simulink model "CF025A_GmFctDiArbn"  (R2013b)
settings: Solver=FixedStepDiscrete  SolverMode=SingleTasking  StartTime=0.0  StopTime=60  FixedStep=0.002  RelTol=1e-3
values from neighbouring files (symbols this model uses):
  GmFctDiArbnEotHwAgThd = DataDict.Calibration    [CF025A_GmFctDiArbn_DataDict.m]
  GmFctDiArbnEotTi = DataDict.Calibration    [CF025A_GmFctDiArbn_DataDict.m]
  GmFctDiArbnOnCentrHwAgThd = DataDict.Calibration    [CF025A_GmFctDiArbn_DataDict.m]
  GmFctDiArbnOnCentrHwTqThd = DataDict.Calibration    [CF025A_GmFctDiArbn_DataDict.m]
  GmFctDiArbnOnCentrTi = DataDict.Calibration    [CF025A_GmFctDiArbn_DataDict.m]
  GmFctDiArbnSrvTi = DataDict.Calibration    [CF025A_GmFctDiArbn_DataDict.m]
  MICROSECTOSEC_ULS_F32 = DataDict.Constant    [CF025A_GmFctDiArbn_DataDict.m]
  ZEROHWAG_HWDEG_F32 = DataDict.Constant    [CF025A_GmFctDiArbn_DataDict.m]
undefined symbols (not defined in the file or in its folder): GmFctDiArbnSts1, LoaSt1
libraries: simulink x7, FixdToFloat x4
(part 3 of 3)

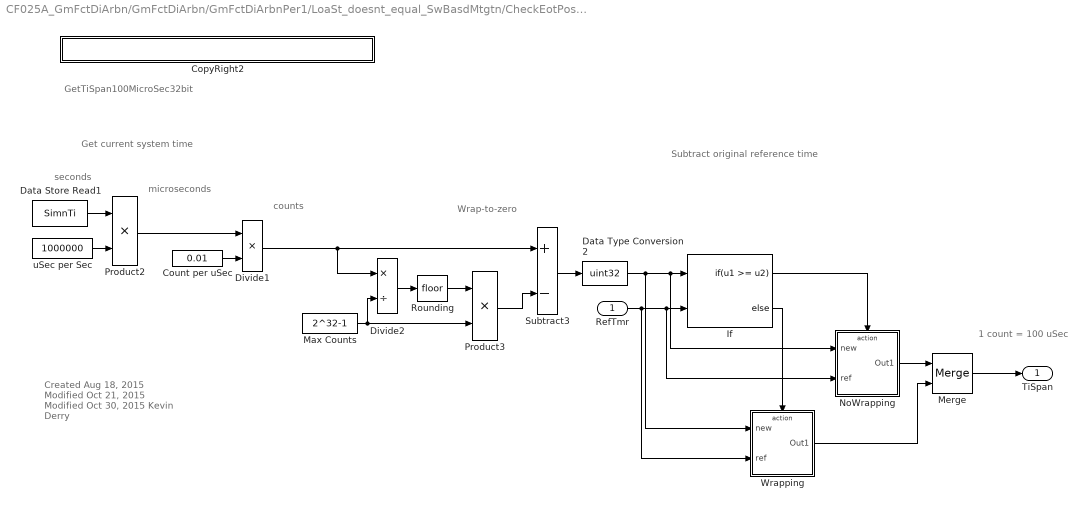
== system CF025A_GmFctDiArbn/GmFctDiArbn/GmFctDiArbnPer1/LoaSt_doesnt_equal_SwBasdMtgtn/CheckEotPosInRange/InProc/InRangeCwDirection/InCwEotElpdTi/ElpdTi_Check/GetTiSpan100MicroSec32bit ==
  note: Created Aug 18, 2015
      | Modified Oct 21, 2015
      | Modified Oct 30, 2015
      | Kevin Derry
  note: GetTiSpan100MicroSec32bit
  note: Get current system time
  note: 1 count = 100 uSec
  note: Wrap-to-zero
  note: counts
  note: microseconds
  note: seconds
  note: Subtract original reference time
  RefTmr : Inport
  CopyRight2 : Subsystem  Description=|  mask(Copyright Information){none=on}
      | Copyright info block.                                               
      |                                                                     
      | Place copyright information at the top of every subsystem in design.
      mask prompts: none "No parameters"
      mask help: Place copyright information at the top of every subsystem in design.
      mask Display:
      | NxtrConf = 'Nexteer Confidential';
      | 
      | sys = bdroot; %handle for the current model ("system")
      | first = get_param(sys,'Created');
      | if(isempty(first))
      |     first = datestr(now,'yyyy');
      | else
      |     first = first(end-3:end);  %year is last four digits
      | end
      | 
      | last = get_param(sys,'LastModifiedDate');
      | if isempty(last)
      |     last = datestr(now,'yyyy');
      | else
      |     last = last(end-3:end);
      | end
      | 
      | if strcmp(first,last)
      |     fprintf('%s -- Copyright %s Nexteer',NxtrConf,first)
      | else
      |     fprintf('%s -- %s%s- %s Nexteer',NxtrConf,char(169),first,last)
      | end
  Count per uSec : Constant  Value=0.01
  Data Store Read1 : DataStoreRead  DataStoreName=SimnTi
  Data Type Conversion2 : DataTypeConversion  OutDataTypeStr=uint32
  Divide1 : Product  Inputs=**
  Divide2 : Product  Inputs=*/
  If : If  NumInputs=2  IfExpression=u1 >= u2
  Max Counts : Constant  Value=2^32-1
  Merge : Merge
  NoWrapping : Subsystem  TreatAsAtomicUnit=on
  Product2 : Product
  Product3 : Product
  Rounding : Rounding
  Subtract3 : Sum  Inputs=+-
  Wrapping : Subsystem  TreatAsAtomicUnit=on
  uSec per Sec : Constant  Value=1000000
  TiSpan : Outport
  wires:
  Data Type Conversion2/1 -> Wrapping/1(new), NoWrapping/1(new), If/1
  RefTmr/1 -> Wrapping/2(ref), NoWrapping/2(ref), If/2
  Merge/1 -> TiSpan/1
  uSec per Sec/1 -> Product2/2
  Count per uSec/1 -> Divide1/2
  Data Store Read1/1 -> Product2/1
  Product2/1 -> Divide1/1
  Divide1/1 -> Subtract3/1, Divide2/1
  Max Counts/1 -> Product3/2, Divide2/2
  Divide2/1 -> Rounding/1
  Rounding/1 -> Product3/1
  Subtract3/1 -> Data Type Conversion2/1
  Product3/1 -> Subtract3/2
  If/1 -> NoWrapping/Action
  If/2 -> Wrapping/Action
  NoWrapping/1(Out1) -> Merge/1
  Wrapping/1(Out1) -> Merge/2

== system CF025A_GmFctDiArbn/GmFctDiArbn/GmFctDiArbnPer1/LoaSt_doesnt_equal_SwBasdMtgtn/CheckEotPosInRange/InProc/InRangeCwDirection/InCwEotElpdTi/ElpdTi_Start/Copyright1 ==

== system CF025A_GmFctDiArbn/GmFctDiArbn/GmFctDiArbnPer1/LoaSt_doesnt_equal_SwBasdMtgtn/CheckEotPosInRange/InProc/InRangeCwDirection/InCwEotElpdTi/ElpdTi_Start/GetRefTmr100MicroSec32bit ==
  note: 1 count = 100 uSec
  note: seconds
  note: microseconds
  note: counts
  note: Wrap-to-zero
  note: GetRefTmr100MicroSec32bit
  note: Created Aug 18, 2015
      | Modified Oct 21, 2015
      | Modified Oct 30, 2015
      | Kevin Derry
  CopyRight2 : Subsystem  Description=|  mask(Copyright Information){none=on}
      | Copyright info block.                                               
      |                                                                     
      | Place copyright information at the top of every subsystem in design.
      mask prompts: none "No parameters"
      mask help: Place copyright information at the top of every subsystem in design.
      mask Display:
      | NxtrConf = 'Nexteer Confidential';
      | 
      | sys = bdroot; %handle for the current model ("system")
      | first = get_param(sys,'Created');
      | if(isempty(first))
      |     first = datestr(now,'yyyy');
      | else
      |     first = first(end-3:end);  %year is last four digits
      | end
      | 
      | last = get_param(sys,'LastModifiedDate');
      | if isempty(last)
      |     last = datestr(now,'yyyy');
      | else
      |     last = last(end-3:end);
      | end
      | 
      | if strcmp(first,last)
      |     fprintf('%s -- Copyright %s Nexteer',NxtrConf,first)
      | else
      |     fprintf('%s -- %s%s- %s Nexteer',NxtrConf,char(169),first,last)
      | end
  Count per uSec : Constant  Value=0.01
  Data Store Read1 : DataStoreRead  DataStoreName=SimnTi
  Data Type Conversion1 : DataTypeConversion  OutDataTypeStr=uint32
  Divide1 : Product  Inputs=**
  Divide2 : Product  Inputs=*/
  Max Counts : Constant  Value=2^32-1
  Product1 : Product
  Product2 : Product
  Rounding : Rounding
  Subtract1 : Sum  Inputs=+-
  uSec per Sec : Constant  Value=1000000
  RefTmr : Outport
  wires:
  Product2/1 -> Subtract1/2
  Subtract1/1 -> Data Type Conversion1/1
  Rounding/1 -> Product2/1
  Divide2/1 -> Rounding/1
  Max Counts/1 -> Divide2/2, Product2/2
  Divide1/1 -> Divide2/1, Subtract1/1
  Product1/1 -> Divide1/1
  Count per uSec/1 -> Divide1/2
  uSec per Sec/1 -> Product1/2
  Data Type Conversion1/1 -> RefTmr/1
  Data Store Read1/1 -> Product1/1

== system CF025A_GmFctDiArbn/GmFctDiArbn/GmFctDiArbnPer1/LoaSt_doesnt_equal_SwBasdMtgtn/CheckEotPosInRange/InProc/InRangeCwDirection/InCwEotElpdTi/ElpdTi_Zero/Copyright1 ==

== system CF025A_GmFctDiArbn/GmFctDiArbn/GmFctDiArbnPer1/LoaSt_doesnt_equal_SwBasdMtgtn/CheckHwTqZeroAndHwAgZero/IfBothEotElpdTimeMet/OnCentrElpdTi/ElpdTi_Check/GetTiSpan100MicroSec32bit/CopyRight2 ==

== system CF025A_GmFctDiArbn/GmFctDiArbn/GmFctDiArbnPer1/LoaSt_doesnt_equal_SwBasdMtgtn/CheckHwTqZeroAndHwAgZero/IfBothEotElpdTimeMet/OnCentrElpdTi/ElpdTi_Check/GetTiSpan100MicroSec32bit/NoWrapping ==
  new : Inport
  ref : Inport  Port=2
  Action Port : ActionPort  ActionType=then
  CopyRight2 : Subsystem  Description=|  mask(Copyright Information){none=on}
      | Copyright info block.                                               
      |                                                                     
      | Place copyright information at the top of every subsystem in design.
      mask prompts: none "No parameters"
      mask help: Place copyright information at the top of every subsystem in design.
      mask Display:
      | NxtrConf = 'Nexteer Confidential';
      | 
      | sys = bdroot; %handle for the current model ("system")
      | first = get_param(sys,'Created');
      | if(isempty(first))
      |     first = datestr(now,'yyyy');
      | else
      |     first = first(end-3:end);  %year is last four digits
      | end
      | 
      | last = get_param(sys,'LastModifiedDate');
      | if isempty(last)
      |     last = datestr(now,'yyyy');
      | else
      |     last = last(end-3:end);
      | end
      | 
      | if strcmp(first,last)
      |     fprintf('%s -- Copyright %s Nexteer',NxtrConf,first)
      | else
      |     fprintf('%s -- %s%s- %s Nexteer',NxtrConf,char(169),first,last)
      | end
  Subtract1 : Sum  Inputs=+-
  Out1 : Outport
  wires:
  Subtract1/1 -> Out1/1
  new/1 -> Subtract1/1
  ref/1 -> Subtract1/2

== system CF025A_GmFctDiArbn/GmFctDiArbn/GmFctDiArbnPer1/LoaSt_doesnt_equal_SwBasdMtgtn/CheckHwTqZeroAndHwAgZero/IfBothEotElpdTimeMet/OnCentrElpdTi/ElpdTi_Check/GetTiSpan100MicroSec32bit/Wrapping ==
  new : Inport
  ref : Inport  Port=2
  Action Port : ActionPort  ActionType=else
  CopyRight2 : Subsystem  Description=|  mask(Copyright Information){none=on}
      | Copyright info block.                                               
      |                                                                     
      | Place copyright information at the top of every subsystem in design.
      mask prompts: none "No parameters"
      mask help: Place copyright information at the top of every subsystem in design.
      mask Display:
      | NxtrConf = 'Nexteer Confidential';
      | 
      | sys = bdroot; %handle for the current model ("system")
      | first = get_param(sys,'Created');
      | if(isempty(first))
      |     first = datestr(now,'yyyy');
      | else
      |     first = first(end-3:end);  %year is last four digits
      | end
      | 
      | last = get_param(sys,'LastModifiedDate');
      | if isempty(last)
      |     last = datestr(now,'yyyy');
      | else
      |     last = last(end-3:end);
      | end
      | 
      | if strcmp(first,last)
      |     fprintf('%s -- Copyright %s Nexteer',NxtrConf,first)
      | else
      |     fprintf('%s -- %s%s- %s Nexteer',NxtrConf,char(169),first,last)
      | end
  Max Counts : Constant  Value=2^32-1  OutDataTypeStr=uint32
  Subtract1 : Sum  Inputs=+-+
  Out1 : Outport
  wires:
  Subtract1/1 -> Out1/1
  Max Counts/1 -> Subtract1/1
  ref/1 -> Subtract1/2
  new/1 -> Subtract1/3

== system CF025A_GmFctDiArbn/GmFctDiArbn/GmFctDiArbnPer1/LoaSt_doesnt_equal_SwBasdMtgtn/CheckHwTqZeroAndHwAgZero/IfBothEotElpdTimeMet/OnCentrElpdTi/ElpdTi_Start/GetRefTmr100MicroSec32bit/CopyRight2 ==

== system CF025A_GmFctDiArbn/GmFctDiArbn/GmFctDiArbnPer1/LoaSt_doesnt_equal_SwBasdMtgtn/CheckEotPosInRange/InProc/InRangeCcwDirection/InCcwEotElpdTi/ElpdTi_Check/GetTiSpan100MicroSec32bit/CopyRight2 ==

== system CF025A_GmFctDiArbn/GmFctDiArbn/GmFctDiArbnPer1/LoaSt_doesnt_equal_SwBasdMtgtn/CheckEotPosInRange/InProc/InRangeCcwDirection/InCcwEotElpdTi/ElpdTi_Check/GetTiSpan100MicroSec32bit/NoWrapping ==
  new : Inport
  ref : Inport  Port=2
  Action Port : ActionPort  ActionType=then
  CopyRight2 : Subsystem  Description=|  mask(Copyright Information){none=on}
      | Copyright info block.                                               
      |                                                                     
      | Place copyright information at the top of every subsystem in design.
      mask prompts: none "No parameters"
      mask help: Place copyright information at the top of every subsystem in design.
      mask Display:
      | NxtrConf = 'Nexteer Confidential';
      | 
      | sys = bdroot; %handle for the current model ("system")
      | first = get_param(sys,'Created');
      | if(isempty(first))
      |     first = datestr(now,'yyyy');
      | else
      |     first = first(end-3:end);  %year is last four digits
      | end
      | 
      | last = get_param(sys,'LastModifiedDate');
      | if isempty(last)
      |     last = datestr(now,'yyyy');
      | else
      |     last = last(end-3:end);
      | end
      | 
      | if strcmp(first,last)
      |     fprintf('%s -- Copyright %s Nexteer',NxtrConf,first)
      | else
      |     fprintf('%s -- %s%s- %s Nexteer',NxtrConf,char(169),first,last)
      | end
  Subtract1 : Sum  Inputs=+-
  Out1 : Outport
  wires:
  ref/1 -> Subtract1/2
  new/1 -> Subtract1/1
  Subtract1/1 -> Out1/1

== system CF025A_GmFctDiArbn/GmFctDiArbn/GmFctDiArbnPer1/LoaSt_doesnt_equal_SwBasdMtgtn/CheckEotPosInRange/InProc/InRangeCcwDirection/InCcwEotElpdTi/ElpdTi_Check/GetTiSpan100MicroSec32bit/Wrapping ==
  new : Inport
  ref : Inport  Port=2
  Action Port : ActionPort  ActionType=else
  CopyRight2 : Subsystem  Description=|  mask(Copyright Information){none=on}
      | Copyright info block.                                               
      |                                                                     
      | Place copyright information at the top of every subsystem in design.
      mask prompts: none "No parameters"
      mask help: Place copyright information at the top of every subsystem in design.
      mask Display:
      | NxtrConf = 'Nexteer Confidential';
      | 
      | sys = bdroot; %handle for the current model ("system")
      | first = get_param(sys,'Created');
      | if(isempty(first))
      |     first = datestr(now,'yyyy');
      | else
      |     first = first(end-3:end);  %year is last four digits
      | end
      | 
      | last = get_param(sys,'LastModifiedDate');
      | if isempty(last)
      |     last = datestr(now,'yyyy');
      | else
      |     last = last(end-3:end);
      | end
      | 
      | if strcmp(first,last)
      |     fprintf('%s -- Copyright %s Nexteer',NxtrConf,first)
      | else
      |     fprintf('%s -- %s%s- %s Nexteer',NxtrConf,char(169),first,last)
      | end
  Max Counts : Constant  Value=2^32-1  OutDataTypeStr=uint32
  Subtract1 : Sum  Inputs=+-+
  Out1 : Outport
  wires:
  new/1 -> Subtract1/3
  ref/1 -> Subtract1/2
  Max Counts/1 -> Subtract1/1
  Subtract1/1 -> Out1/1

== system CF025A_GmFctDiArbn/GmFctDiArbn/GmFctDiArbnPer1/LoaSt_doesnt_equal_SwBasdMtgtn/CheckEotPosInRange/InProc/InRangeCcwDirection/InCcwEotElpdTi/ElpdTi_Start/GetRefTmr100MicroSec32bit/CopyRight2 ==

== system CF025A_GmFctDiArbn/GmFctDiArbn/GmFctDiArbnPer1/LoaSt_doesnt_equal_SwBasdMtgtn/CheckEotPosInRange/InProc/InRangeCwDirection/InCwEotElpdTi/ElpdTi_Check/GetTiSpan100MicroSec32bit/CopyRight2 ==

== system CF025A_GmFctDiArbn/GmFctDiArbn/GmFctDiArbnPer1/LoaSt_doesnt_equal_SwBasdMtgtn/CheckEotPosInRange/InProc/InRangeCwDirection/InCwEotElpdTi/ElpdTi_Check/GetTiSpan100MicroSec32bit/NoWrapping ==
  new : Inport
  ref : Inport  Port=2
  Action Port : ActionPort  ActionType=then
  CopyRight2 : Subsystem  Description=|  mask(Copyright Information){none=on}
      | Copyright info block.                                               
      |                                                                     
      | Place copyright information at the top of every subsystem in design.
      mask prompts: none "No parameters"
      mask help: Place copyright information at the top of every subsystem in design.
      mask Display:
      | NxtrConf = 'Nexteer Confidential';
      | 
      | sys = bdroot; %handle for the current model ("system")
      | first = get_param(sys,'Created');
      | if(isempty(first))
      |     first = datestr(now,'yyyy');
      | else
      |     first = first(end-3:end);  %year is last four digits
      | end
      | 
      | last = get_param(sys,'LastModifiedDate');
      | if isempty(last)
      |     last = datestr(now,'yyyy');
      | else
      |     last = last(end-3:end);
      | end
      | 
      | if strcmp(first,last)
      |     fprintf('%s -- Copyright %s Nexteer',NxtrConf,first)
      | else
      |     fprintf('%s -- %s%s- %s Nexteer',NxtrConf,char(169),first,last)
      | end
  Subtract1 : Sum  Inputs=+-
  Out1 : Outport
  wires:
  Subtract1/1 -> Out1/1
  new/1 -> Subtract1/1
  ref/1 -> Subtract1/2

== system CF025A_GmFctDiArbn/GmFctDiArbn/GmFctDiArbnPer1/LoaSt_doesnt_equal_SwBasdMtgtn/CheckEotPosInRange/InProc/InRangeCwDirection/InCwEotElpdTi/ElpdTi_Check/GetTiSpan100MicroSec32bit/Wrapping ==
  new : Inport
  ref : Inport  Port=2
  Action Port : ActionPort  ActionType=else
  CopyRight2 : Subsystem  Description=|  mask(Copyright Information){none=on}
      | Copyright info block.                                               
      |                                                                     
      | Place copyright information at the top of every subsystem in design.
      mask prompts: none "No parameters"
      mask help: Place copyright information at the top of every subsystem in design.
      mask Display:
      | NxtrConf = 'Nexteer Confidential';
      | 
      | sys = bdroot; %handle for the current model ("system")
      | first = get_param(sys,'Created');
      | if(isempty(first))
      |     first = datestr(now,'yyyy');
      | else
      |     first = first(end-3:end);  %year is last four digits
      | end
      | 
      | last = get_param(sys,'LastModifiedDate');
      | if isempty(last)
      |     last = datestr(now,'yyyy');
      | else
      |     last = last(end-3:end);
      | end
      | 
      | if strcmp(first,last)
      |     fprintf('%s -- Copyright %s Nexteer',NxtrConf,first)
      | else
      |     fprintf('%s -- %s%s- %s Nexteer',NxtrConf,char(169),first,last)
      | end
  Max Counts : Constant  Value=2^32-1  OutDataTypeStr=uint32
  Subtract1 : Sum  Inputs=+-+
  Out1 : Outport
  wires:
  Subtract1/1 -> Out1/1
  Max Counts/1 -> Subtract1/1
  ref/1 -> Subtract1/2
  new/1 -> Subtract1/3

== system CF025A_GmFctDiArbn/GmFctDiArbn/GmFctDiArbnPer1/LoaSt_doesnt_equal_SwBasdMtgtn/CheckEotPosInRange/InProc/InRangeCwDirection/InCwEotElpdTi/ElpdTi_Start/GetRefTmr100MicroSec32bit/CopyRight2 ==

== system CF025A_GmFctDiArbn/GmFctDiArbn/GmFctDiArbnPer1/LoaSt_doesnt_equal_SwBasdMtgtn/CheckHwTqZeroAndHwAgZero/IfBothEotElpdTimeMet/OnCentrElpdTi/ElpdTi_Check/GetTiSpan100MicroSec32bit/NoWrapping/CopyRight2 ==

== system CF025A_GmFctDiArbn/GmFctDiArbn/GmFctDiArbnPer1/LoaSt_doesnt_equal_SwBasdMtgtn/CheckHwTqZeroAndHwAgZero/IfBothEotElpdTimeMet/OnCentrElpdTi/ElpdTi_Check/GetTiSpan100MicroSec32bit/Wrapping/CopyRight2 ==

== system CF025A_GmFctDiArbn/GmFctDiArbn/GmFctDiArbnPer1/LoaSt_doesnt_equal_SwBasdMtgtn/CheckEotPosInRange/InProc/InRangeCcwDirection/InCcwEotElpdTi/ElpdTi_Check/GetTiSpan100MicroSec32bit/NoWrapping/CopyRight2 ==

== system CF025A_GmFctDiArbn/GmFctDiArbn/GmFctDiArbnPer1/LoaSt_doesnt_equal_SwBasdMtgtn/CheckEotPosInRange/InProc/InRangeCcwDirection/InCcwEotElpdTi/ElpdTi_Check/GetTiSpan100MicroSec32bit/Wrapping/CopyRight2 ==

== system CF025A_GmFctDiArbn/GmFctDiArbn/GmFctDiArbnPer1/LoaSt_doesnt_equal_SwBasdMtgtn/CheckEotPosInRange/InProc/InRangeCwDirection/InCwEotElpdTi/ElpdTi_Check/GetTiSpan100MicroSec32bit/NoWrapping/CopyRight2 ==

== system CF025A_GmFctDiArbn/GmFctDiArbn/GmFctDiArbnPer1/LoaSt_doesnt_equal_SwBasdMtgtn/CheckEotPosInRange/InProc/InRangeCwDirection/InCwEotElpdTi/ElpdTi_Check/GetTiSpan100MicroSec32bit/Wrapping/CopyRight2 ==
